simulink model "noisesSim"  (R2015a)
settings: Solver=ode45  StartTime=0.0  StopTime=25/f0  RelTol=1e-3
model workspace (MATLAB code in the model file):
  | f0=1;
  | w0=2*pi*f0;
  | ts=1/(10*f0)
libraries: simulink x1, simulink_extras x1
settings Model: Creator=mainster  LastModifiedBy=mainster

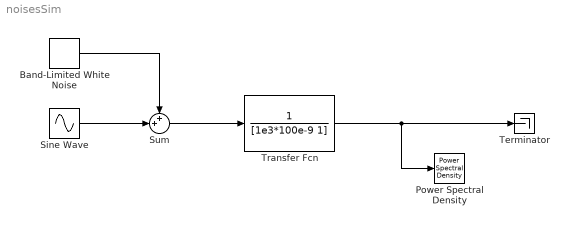
== system noisesSim ==
  Band-Limited White Noise : simulink/Sources/Band-Limited White Noise  Cov=[0.01]  Ts=ts  seed=[23341]
  Power Spectral Density : simulink_extras/Additional Sinks/Power Spectral Density  npts=128  fftpts=512  HowOften=128  sampleT=ts
  Sine Wave : Sin  Amplitude=10e-3*0  Frequency=w0  SampleTime=0
  Sum : Sum  Inputs=++|
  Terminator : Terminator
  Transfer Fcn : TransferFcn  Denominator=[1e3*100e-9 1]
  wires:
  Band-Limited White Noise/1 -> Sum/1
  Sine Wave/1 -> Sum/2
  Sum/1 -> Transfer Fcn/1
  Transfer Fcn/1 -> Power Spectral Density/1, Terminator/1
